simulink library "INT_RngMod_TrqSpdCrv"  (R2016b)
settings: Solver=VariableStepAuto  StartTime=0.0  StopTime=10.0  RelTol=1e-3
settings Model: Creator=Administrator  LastModifiedBy=Administrator

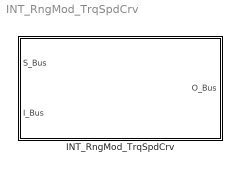
== system INT_RngMod_TrqSpdCrv ==
  INT_RngMod_TrqSpdCrv : Subsystem

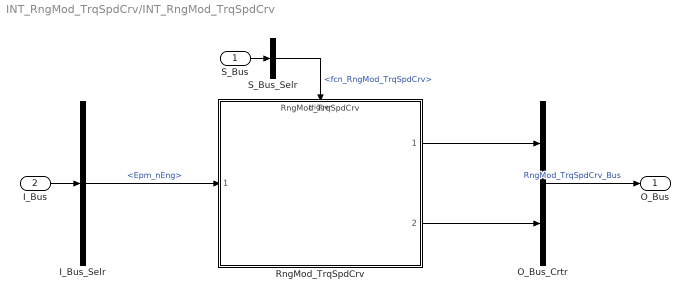
== system INT_RngMod_TrqSpdCrv/INT_RngMod_TrqSpdCrv ==
  S_Bus : Inport
  I_Bus : Inport  Port=2
  I_Bus_Selr : BusSelector  OutputSignals=Epm_nEng
  O_Bus_Crtr : BusCreator  Inputs=2
  RngMod_TrqSpdCrv : ModelReference  ModelNameDialog=RngMod_TrqSpdCrv  SimulationMode=Normal  ModelReferenceVersion=1.2  TriggerPortName=function  TriggerPortTriggerType=function-call  TriggerPortStatesWhenEnabling=held
  S_Bus_Selr : BusSelector  OutputSignals=fcn_RngMod_TrqSpdCrv
  O_Bus : Outport
  wires:
  S_Bus_Selr/1 -> RngMod_TrqSpdCrv/Trigger  "<fcn_RngMod_TrqSpdCrv>"
  S_Bus/1 -> S_Bus_Selr/1
  I_Bus/1 -> I_Bus_Selr/1
  I_Bus_Selr/1 -> RngMod_TrqSpdCrv/1  "<Epm_nEng>"
  O_Bus_Crtr/1 -> O_Bus/1  "RngMod_TrqSpdCrv_Bus"
  RngMod_TrqSpdCrv/1 -> O_Bus_Crtr/1
  RngMod_TrqSpdCrv/2 -> O_Bus_Crtr/2
